simulink model "sampleModel2060"  (R2023a)
settings: Solver=VariableStepAuto  StartTime=0.0  StopTime=10.0  RelTol=1e-3
libraries: hdlsllib x10
settings Model: Creator=user1  LastModifiedBy=user1

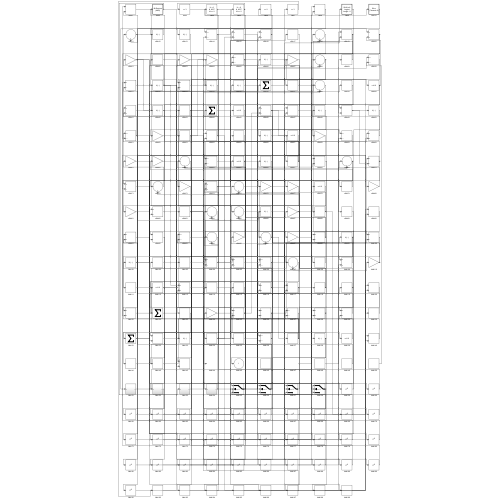
[thumbnail: Simulink's stored preview of the top-level diagram]
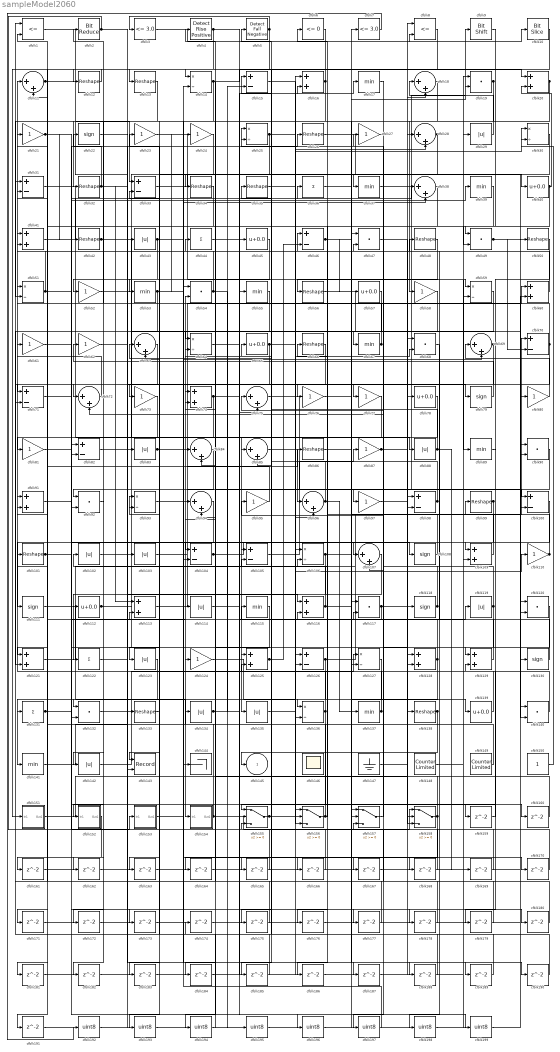
== system sampleModel2060 ==
  cfblk1 : RelationalOperator  Operator=<=  OutDataTypeStr=boolean  InputSameDT=off
  cfblk10 : hdlsllib/Logic and Bit Operations/Bit Slice  lidx=7  ridx=0
  cfblk{15,31,33,46,70..71,82,98,100,104..105,126} (12 alike) : Sum  Inputs=+-
  cfblk{12..13,26,32,34..35,42,48,50,56,66,86,99,101,133,138} (16 alike) : Reshape
  cfblk{29,43,83,88,102..103,114,119,123,134..135,142} (12 alike) : Abs  SaturateOnIntegerOverflow=off
  cfblk{14,25,30,51,59,64,93,106,127,136} (10 alike) : Product  Inputs=*/  RndMeth=Zero  SaturateOnIntegerOverflow=on
  cfblk{11,18,28,38,63,69,72,75,84..85,94,96,107} (13 alike) : Sum  Inputs=|++
  cfblk{22,79,108,111,118,130} (6 alike) : Signum
  cfblk{16,20,41,60,74,91,109,113,116,121,125,128..129} (13 alike) : Sum
  cfblk{21,23..24,27,52,58,61..62,73,76..77,80..81,87,95,97,110,124} (18 alike) : Gain
  cfblk{40,45,57,65,78,112,139} (7 alike) : Bias  Bias=0.0  SaturateOnIntegerOverflow=off
  cfblk{17,37,39,53,55,67,89,115,137,141} (10 alike) : MinMax
  cfblk{19,47,49,54,68,90,92,117,120,132,140} (11 alike) : DotProduct  OutDataTypeStr=Inherit: Inherit via internal rule
  cfblk{36,44,122,131} (4 alike) : Sum  Inputs=+
  cfblk143 : Record  FileSettingsInternal="{\"entries\":[{\"content\":{\"excelSettings\":{\"content\":{},\"type\":\"Streamout.ExcelSettings\"}},\"type\":\"Streamout.FileSettingStorage\",\"uuid\":\"\"}],\"packageUris\":[\"http:\\/\\/schema.mathworks.com\\/mf0\\/streamout_blocks\\/R2020a\"],\"version\":\"1.0\"}"  Layout=[1 1]  SignalsInternal="{\"entries\":[{\"content\":{\"signals\":[{\"content\":{\"blockPath\":[],\"dimensions\":[1],\"domain\":\"\",\"lineColor\":\"#a2142f\",\"plots\":[1],\"port\":1,\"signalID\":6360,\"signalName\":\"XY Graph:1\"},\"type\":\"RecordBlkView.Signal\",\"uuid\":\"\"},{\"content\":{\"blockPath\":[],\"dimensions\":[1],\"domain\":\"\",\"lineColor\":\"#139fff\",\"plots\":[1],\"port\":2,\"signalID\":6363,\"signalName\":\"XY Graph:2\"},\"type\":\"RecordBlkView.Signal\",\"uuid\":\"\"}]},\"type\":\"RecordBlkView.InputSignals\",\"uuid\":\"\"}],\"packageUris\":[\"http:\\/\\/schema.mathworks.com\\/mf0\\/streamout_blocks\\/R2020a\"],\"version\":\"1.0\"}"  VisualizationBindings="{\"xyplotplugin\":{\"info\":[{\"series\":[{\"bindingParametersList\":[{\"parameter\":\"X-Axis\",\"signalID\":6360,\"signalName\":\"XY Graph:1\"},{\"parameter\":\"Y-Axis\",\"signalID\":6363,\"signalName\":\"XY Graph:2\"}],\"seriesID\":60653}],\"subplotID\":1}]}}"  CompatibilityTag=XY  st=-1
  cfblk144 : Terminator
  cfblk146 : Scope
      settings: Floating=on
  cfblk147 : Ground
  cfblk148 : hdlsllib/Sources/Counter Limited  uplimit=7  tsamp=-1
  cfblk149 : hdlsllib/Sources/Counter Limited  uplimit=7  tsamp=-1
  cfblk150 : Constant  SampleTime=-1
  cfblk151 : Subsystem
      settings: LibrarySourceBlock=|
      | hdlsllib/Ports &
      | Subsystems/Subsystem
  cfblk152 : Subsystem
      settings: LibrarySourceBlock=|
      | hdlsllib/Ports &
      | Subsystems/Subsystem
  cfblk153 : Subsystem
      settings: LibrarySourceBlock=|
      | hdlsllib/Ports &
      | Subsystems/Subsystem
  cfblk154 : Subsystem
      settings: LibrarySourceBlock=|
      | hdlsllib/Ports &
      | Subsystems/Subsystem
  cfblk{155..158} (4 alike) : Switch  SaturateOnIntegerOverflow=off  InputSameDT=off
  cfblk{159..191} (33 alike) : Delay  SampleTime=1
  cfblk{192..199} (8 alike) : DataTypeConversion  OutDataTypeStr=uint8  SaturateOnIntegerOverflow=off  RndMeth=Floor
  cfblk2 : hdlsllib/Logic and Bit Operations/Bit Reduce  mode=AND
  cfblk3 : hdlsllib/Logic and Bit Operations/Compare To Constant  relop=<=  const=3.0  OutDataTypeStr=boolean
  cfblk4 : hdlsllib/Logic and Bit Operations/Detect Rise Positive  vinit=0  OutDataTypeStr=boolean
  cfblk5 : hdlsllib/Logic and Bit Operations/Detect Fall Negative  vinit=0  OutDataTypeStr=boolean
  cfblk6 : hdlsllib/Logic and Bit Operations/Compare To Zero  relop=<=  OutDataTypeStr=boolean
  cfblk7 : hdlsllib/Logic and Bit Operations/Compare To Constant  relop=<=  const=3.0  OutDataTypeStr=boolean
  cfblk8 : RelationalOperator  Operator=<=  OutDataTypeStr=boolean  InputSameDT=off
  cfblk9 : hdlsllib/Logic and Bit Operations/Bit Shift  mode=Shift Left Logical  N=0
  cfblk145 : Outport  VectorParamsAs1DForOutWhenUnconnected=off
  wires:
  cfblk80/1 -> cfblk69/1
  cfblk139/1 -> cfblk11/1
  cfblk105/1 -> cfblk87/1
  cfblk109/1 -> cfblk75/1
  cfblk37/1 -> cfblk155/1
  cfblk93/1 -> cfblk97/1
  cfblk112/1 -> cfblk40/1, cfblk144/1
  cfblk125/1 -> cfblk15/1, cfblk46/2
  cfblk5/1 -> cfblk3/1, cfblk11/2
  cfblk138/1 -> cfblk165/1, cfblk166/1
  cfblk97/1 -> cfblk10/1
  cfblk158/1 -> cfblk44/1, cfblk164/1, cfblk168/1
  cfblk31/1 -> cfblk135/1
  cfblk116/1 -> cfblk102/1, cfblk99/1
  cfblk81/1 -> cfblk36/1
  cfblk123/1 -> cfblk141/1
  cfblk108/1 -> cfblk51/1
  cfblk121/1 -> cfblk78/1
  cfblk78/1 -> cfblk123/1
  cfblk149/1 -> cfblk54/2
  cfblk101/1 -> cfblk39/1, cfblk25/2
  cfblk20/1 -> cfblk58/1, cfblk127/2
  cfblk47/1 -> cfblk98/2
  cfblk118/1 -> cfblk25/1, cfblk74/2
  cfblk63/1 -> cfblk82/2
  cfblk127/1 -> cfblk132/1
  cfblk111/1 -> cfblk154/1(In1)
  cfblk141/1 -> cfblk103/1
  cfblk18/1 -> cfblk32/1
  cfblk86/1 -> cfblk139/1
  cfblk119/1 -> cfblk95/1, cfblk158/3
  cfblk50/1 -> cfblk109/1
  cfblk29/1 -> cfblk18/1
  cfblk42/1 -> cfblk126/1, cfblk182/1
  cfblk11/1 -> cfblk71/1, cfblk33/1
  cfblk9/1 -> cfblk49/1
  cfblk19/1 -> cfblk52/1, cfblk104/2
  cfblk10/1 -> cfblk85/1
  cfblk132/1 -> cfblk45/1
  cfblk53/1 -> cfblk69/2, cfblk24/1, cfblk131/1
  cfblk79/1 -> cfblk62/1
  cfblk83/1 -> cfblk88/1, cfblk156/3, cfblk170/1
  cfblk155/1 -> cfblk65/1, cfblk30/2, cfblk125/2, cfblk115/1, cfblk110/1
  cfblk82/1 -> cfblk26/1
  cfblk55/1 -> cfblk132/2
  cfblk103/1 -> cfblk8/1
  cfblk13/1 -> cfblk51/2
  cfblk41/1 -> cfblk9/1
  cfblk44/1 -> cfblk77/1
  cfblk100/1 -> cfblk129/1
  cfblk87/1 -> cfblk138/1, cfblk167/1
  cfblk12/1 -> cfblk151/1(In1)
  cfblk126/1 -> cfblk70/1, cfblk152/1(In1)
  cfblk60/1 -> cfblk35/1
  cfblk59/1 -> cfblk81/1
  cfblk142/1 -> cfblk84/1
  cfblk6/1 -> cfblk121/1
  cfblk61/1 -> cfblk108/1
  cfblk140/1 -> cfblk106/2
  cfblk1/1 -> cfblk133/1
  cfblk57/1 -> cfblk121/2
  cfblk72/1 -> cfblk61/1
  cfblk23/1 -> cfblk89/1
  cfblk88/1 -> cfblk64/2, cfblk169/1
  cfblk133/1 -> cfblk93/1
  cfblk156/1 -> cfblk66/1, cfblk74/1, cfblk91/2
  cfblk4/1 -> cfblk12/1, cfblk188/1
  cfblk35/1 -> cfblk59/1
  cfblk96/1 -> cfblk63/1, cfblk137/1
  cfblk33/1 -> cfblk37/1
  cfblk32/1 -> cfblk22/1, cfblk76/1, cfblk113/1, cfblk116/1
  cfblk69/1 -> cfblk136/1, cfblk71/2
  cfblk70/1 -> cfblk84/2, cfblk23/1
  cfblk74/1 -> cfblk55/1, cfblk92/2, cfblk17/1
  cfblk3/1 -> cfblk8/2
  cfblk8/1 -> cfblk13/1
  cfblk150/1 -> cfblk30/1
  cfblk26/1 -> cfblk50/1
  cfblk85/1 -> cfblk96/1
  cfblk104/1 -> cfblk107/1, cfblk16/2
  cfblk102/1 -> cfblk43/1
  cfblk64/1 -> cfblk79/1
  cfblk147/1 -> cfblk118/1
  cfblk135/1 -> cfblk28/2
  cfblk99/1 -> cfblk142/1, cfblk143/2
  cfblk106/1 -> cfblk122/1, cfblk60/1
  cfblk151/1(Out1) -> cfblk18/2
  cfblk137/1 -> cfblk124/1, cfblk6/1, cfblk5/1
  cfblk51/1 -> cfblk41/2, cfblk177/1
  cfblk75/1 -> cfblk100/1
  cfblk52/1 -> cfblk130/1
  cfblk154/1(Out1) -> cfblk158/1, cfblk33/2
  cfblk24/1 -> cfblk143/1
  cfblk2/1 -> cfblk153/1(In1), cfblk128/2
  cfblk94/1 -> cfblk111/1
  cfblk130/1 -> cfblk101/1
  cfblk39/1 -> cfblk64/1
  cfblk157/1 -> cfblk47/2
  cfblk40/1 -> cfblk49/2, cfblk72/1, cfblk20/2
  cfblk95/1 -> cfblk31/2
  cfblk134/1 -> cfblk119/1, cfblk15/2, cfblk117/2
  cfblk17/1 -> cfblk107/2
  cfblk124/1 -> cfblk156/2
  cfblk27/1 -> cfblk67/1
  cfblk110/1 -> cfblk41/1, cfblk46/1
  cfblk49/1 -> cfblk80/1, cfblk70/2
  cfblk148/1 -> cfblk29/1
  cfblk16/1 -> cfblk14/1, cfblk53/1
  cfblk36/1 -> cfblk19/2
  cfblk15/1 -> cfblk136/2
  cfblk25/1 -> cfblk157/2, cfblk34/1
  cfblk54/1 -> cfblk21/1, cfblk195/1
  cfblk56/1 -> cfblk140/2
  cfblk131/1 -> cfblk158/2, cfblk114/1
  cfblk58/1 -> cfblk145/1
  cfblk117/1 -> cfblk38/1, cfblk116/2
  cfblk65/1 -> cfblk68/2, cfblk193/1
  cfblk67/1 -> cfblk2/1, cfblk4/1
  cfblk14/1 -> cfblk94/2, cfblk20/1, cfblk163/1
  cfblk113/1 -> cfblk86/1
  cfblk28/1 -> cfblk104/1, cfblk185/1
  cfblk45/1 -> cfblk73/1
  cfblk129/1 -> cfblk48/1
  cfblk136/1 -> cfblk91/1, cfblk175/1
  cfblk77/1 -> cfblk105/1
  cfblk98/1 -> cfblk27/1, cfblk72/2
  cfblk46/1 -> cfblk57/1, cfblk176/1, cfblk180/1
  cfblk153/1(Out1) -> cfblk127/1
  cfblk48/1 -> cfblk56/1
  cfblk84/1 -> cfblk92/1
  cfblk43/1 -> cfblk112/1, cfblk38/2, cfblk187/1
  cfblk21/1 -> cfblk125/1, cfblk42/1, cfblk196/1
  cfblk128/1 -> cfblk134/1, cfblk113/2
  cfblk122/1 -> cfblk159/1
  cfblk159/1 -> cfblk129/2
  cfblk62/1 -> cfblk160/1
  cfblk160/1 -> cfblk106/1
  cfblk73/1 -> cfblk161/1
  cfblk161/1 -> cfblk75/2
  cfblk107/1 -> cfblk162/1
  cfblk162/1 -> cfblk96/2
  cfblk163/1 -> cfblk93/2
  cfblk164/1 -> cfblk140/1
  cfblk165/1 -> cfblk82/1
  cfblk166/1 -> cfblk105/2
  cfblk167/1 -> cfblk60/2
  cfblk168/1 -> cfblk16/1
  cfblk169/1 -> cfblk157/1
  cfblk170/1 -> cfblk155/3
  cfblk66/1 -> cfblk171/1
  cfblk171/1 -> cfblk156/1
  cfblk92/1 -> cfblk172/1
  cfblk172/1 -> cfblk98/1
  cfblk91/1 -> cfblk173/1
  cfblk173/1 -> cfblk128/1
  cfblk174/1 -> cfblk100/2
  cfblk175/1 -> cfblk94/1
  cfblk176/1 -> cfblk59/2
  cfblk177/1 -> cfblk31/1
  cfblk71/1 -> cfblk178/1
  cfblk178/1 -> cfblk1/2
  cfblk89/1 -> cfblk179/1
  cfblk179/1 -> cfblk68/1
  cfblk180/1 -> cfblk157/3
  cfblk152/1(Out1) -> cfblk181/1
  cfblk181/1 -> cfblk126/2
  cfblk182/1 -> cfblk14/2
  cfblk30/1 -> cfblk183/1
  cfblk183/1 -> cfblk155/2
  cfblk115/1 -> cfblk184/1
  cfblk184/1 -> cfblk28/1
  cfblk185/1 -> cfblk63/2
  cfblk38/1 -> cfblk186/1
  cfblk186/1 -> cfblk117/1
  cfblk187/1 -> cfblk109/2
  cfblk188/1 -> cfblk47/1
  cfblk22/1 -> cfblk189/1
  cfblk189/1 -> cfblk1/1
  cfblk76/1 -> cfblk190/1
  cfblk190/1 -> cfblk85/2
  cfblk34/1 -> cfblk191/1
  cfblk191/1 -> cfblk19/1
  cfblk7/1 -> cfblk192/1
  cfblk192/1 -> cfblk83/1
  cfblk193/1 -> cfblk7/1
  cfblk90/1 -> cfblk194/1
  cfblk194/1 -> cfblk174/1
  cfblk195/1 -> cfblk90/1
  cfblk196/1 -> cfblk90/2
  cfblk120/1 -> cfblk197/1
  cfblk197/1 -> cfblk54/1
  cfblk68/1 -> cfblk198/1
  cfblk198/1 -> cfblk120/1
  cfblk114/1 -> cfblk199/1
  cfblk199/1 -> cfblk120/2

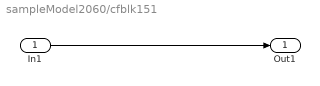
== system sampleModel2060/cfblk151 ==
  In1 : Inport
  Out1 : Outport
  wires:
  In1/1 -> Out1/1

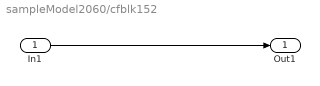
== system sampleModel2060/cfblk152 ==
  In1 : Inport
  Out1 : Outport
  wires:
  In1/1 -> Out1/1

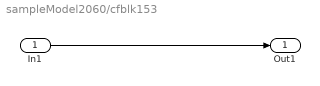
== system sampleModel2060/cfblk153 ==
  In1 : Inport
  Out1 : Outport
  wires:
  In1/1 -> Out1/1

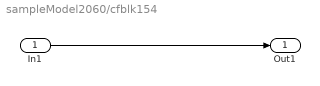
== system sampleModel2060/cfblk154 ==
  In1 : Inport
  Out1 : Outport
  wires:
  In1/1 -> Out1/1
